simulink model "lisan2"  (R2018b)
settings: Solver=VariableStepAuto  StartTime=0.0  StopTime=10.0  RelTol=1e-3
libraries: discretizing x1
settings Model: Creator=QJ-  LastModifiedBy=QJ-

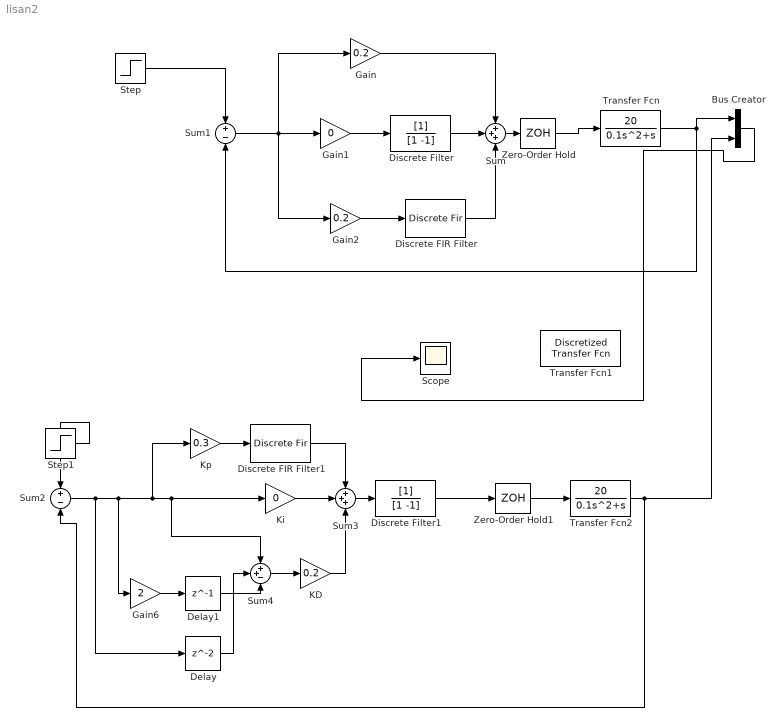
== system lisan2 ==
  Bus Creator : BusCreator  Inputs=3
  Delay : Delay  SampleTime=0.1
  Delay1 : Delay  DelayLength=1  SampleTime=0.1
  Discrete FIR Filter : DiscreteFir  Coefficients=[1 -1]  SampleTime=0.1
  Discrete FIR Filter1 : DiscreteFir  Coefficients=[1 -1]  SampleTime=0.1
  Discrete Filter : DiscreteFilter  Denominator=[1 -1]  SampleTime=0.1
  Discrete Filter1 : DiscreteFilter  Denominator=[1 -1]
  Gain : Gain  Gain=0.2
  Gain1 : Gain  Gain=0
  Gain2 : Gain  Gain=0.2
  Gain6 : Gain  Gain=2
  "KD " : Gain  Gain=0.2
  "Ki " : Gain  Gain=0
  "Kp " : Gain  Gain=0.3
  Scope : Scope
  Step : Step  SampleTime=0.1
  Step1 : Step  SampleTime=0.1
  Sum : Sum  Inputs=+++
  Sum1 : Sum  Inputs=+-
  Sum2 : Sum  Inputs=+-
  Sum3 : Sum  Inputs=+++
  Sum4 : Sum  Inputs=++-
  Transfer Fcn : TransferFcn  Numerator=[20]  Denominator=[0.1 1 0]
  Transfer Fcn1 : discretizing/Discretized Transfer Fcn  Numerator=[20]  Denominator=[0.1 1 0]  AbsTol=auto  SampleTime=0.1  method=zoh  Wc=0
  Transfer Fcn2 : TransferFcn  Numerator=[20]  Denominator=[0.1 1 0]
  Zero-Order Hold : ZeroOrderHold  SampleTime=0.1
  Zero-Order Hold1 : ZeroOrderHold  SampleTime=0.1
  wires:
  Gain/1 -> Sum/1
  Discrete Filter/1 -> Sum/2
  Gain1/1 -> Discrete Filter/1
  Discrete FIR Filter/1 -> Sum/3
  Gain2/1 -> Discrete FIR Filter/1
  Step/1 -> Sum1/1
  Sum1/1 -> Gain2/1, Gain1/1, Gain/1
  Bus Creator/1 -> Scope/1
  Sum/1 -> Zero-Order Hold/1
  Zero-Order Hold/1 -> Transfer Fcn/1
  Transfer Fcn/1 -> Bus Creator/1, Sum1/2
  "Kp "/1 -> Discrete FIR Filter1/1
  Discrete FIR Filter1/1 -> Sum3/1
  "Ki "/1 -> Sum3/2
  "KD "/1 -> Sum3/3
  Sum4/1 -> "KD "/1
  Sum2/1 -> Gain6/1, "Kp "/1, Sum4/1, "Ki "/1, Delay/1
  Step1/1 -> Sum2/1
  Delay/1 -> Sum4/2
  Gain6/1 -> Delay1/1
  Delay1/1 -> Sum4/3
  Zero-Order Hold1/1 -> Transfer Fcn2/1
  Transfer Fcn2/1 -> Bus Creator/3, Sum2/2
  Sum3/1 -> Discrete Filter1/1
  Discrete Filter1/1 -> Zero-Order Hold1/1
